simulink model "ship_location_measurements_model_dynamic"  (R2024b)
settings: Solver=VariableStepAuto  StartTime=0.0  StopTime=300  RelTol=1e-3
InitFcn:
  | dt=1;
settings Model: Creator=Noy Kirshner  LastModifiedBy=danie
settings SolverCC: AlgebraicLoopSolver=TrustRegion
settings RTWCC: GPUComputeCapability=3.5  DLArmComputeVersion=19.05

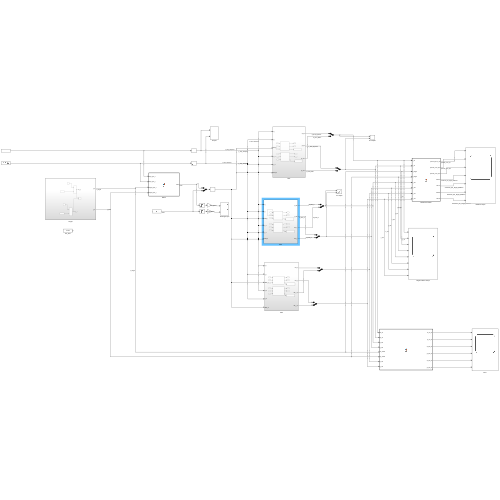
[thumbnail: Simulink's stored preview of the top-level diagram]
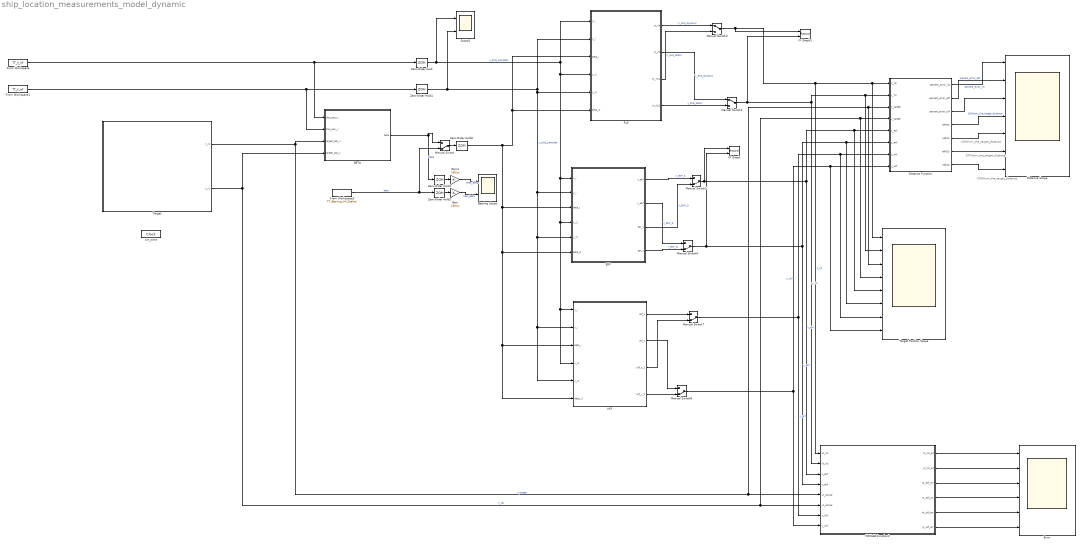
== system ship_location_measurements_model_dynamic ==
  note: -20%from_the_target_distance
  note: 20%from_the_target_distance
  note: -10%from_the_target_distance
  " Bearing Scope" : Scope  NumInputPorts=2
  " Scope1" : Scope  NumInputPorts=2
  BETA : MATLAB Function  TreatAsAtomicUnit=on
  Distance Function : MATLAB Function  TreatAsAtomicUnit=on
  Distance Scope : Scope  NumInputPorts=7
  EKF : Subsystem
  Error : Scope  NumInputPorts=6
      settings: Description=error
  From Workspace : FromWorkspace  VariableName=TT_X_inf  SampleTime=0.001
  From Workspace1 : FromWorkspace  VariableName=TT_Y_inf  SampleTime=0.001
  From Workspace3 : FromWorkspace  VariableName=TT_Bearing_Inf_Scaled
  Gain : Gain  Gain=180/pi
  Gain1 : Gain  Gain=180/pi
  MATLAB Function2 : MATLAB Function  TreatAsAtomicUnit=on
  Manual Switch{,4..7} (5 alike) : ManualSwitch  CurrentSetting=0
  Manual Switch2 : ManualSwitch
  Manual Switch3 : ManualSwitch
  RLS : Subsystem
  Target : Subsystem
  Target Position Scope : Scope  NumInputPorts=8
  UKF : Subsystem
  XY Graph : Record  FileSettingsInternal="{\"entries\":[{\"content\":{\"excelSettings\":{\"content\":{},\"type\":\"Streamout.ExcelSettings\"}},\"type\":\"Streamout.FileSettingStorage\",\"uuid\":\"\"}],\"packageUris\":[\"http:\\/\\/schema.mathworks.com\\/mf0\\/streamout_blocks\\/R2020a\"],\"version\":\"1.0\"}"  Layout=[1 1]  SignalsInternal="{\"entries\":[{\"content\":{\"signals\":[{\"content\":{\"blockPath\":[],\"dimensions\":[1],\"domain\":\"\",\"lineColor\":\"#a2142f\",\"plots\":[ 1 ],\"port\":1,\"signalID\":1,\"signalName\":\"x_ekf\"},\"type\":\"RecordBlkView.Signal\",\"uuid\":\"\"},{\"content\":{\"blockPath\":[],\"dimensions\":[1],\"domain\":\"\",\"lineColor\":\"#139fff\",\"plots\":[ 1 ],\"port\":2,\"signalID\":2,\"signalName\":\"y_ekf\"},\"type\":\"RecordBlkView.Signal\",\"uuid\":\"\"}]},\"type\":\"RecordBlkView.InputSignals\",\"uuid\":\"\"}],\"packageUris\":[\"http:\\/\\/schema.mathworks.com\\/mf0\\/streamout_blocks\\/R2020a\"],\"version\":\"1.0\"}"  VisualizationBindings="{\"xyplotplugin\":{\"info\":[{\"series\":[{\"bindingParametersList\":[{\"parameter\":\"X-Axis\",\"signalID\":1,\"signalName\":\"x_ekf\"},{\"parameter\":\"Y-Axis\",\"signalID\":2,\"signalName\":\"y_ekf\"}],\"seriesID\":0}],\"subplotID\":1}]}}"  CompatibilityTag=XY
  XY Graph1 : Record  FileSettingsInternal="{\"entries\":[{\"content\":{\"excelSettings\":{\"content\":{},\"type\":\"Streamout.ExcelSettings\"}},\"type\":\"Streamout.FileSettingStorage\",\"uuid\":\"\"}],\"packageUris\":[\"http:\\/\\/schema.mathworks.com\\/mf0\\/streamout_blocks\\/R2020a\"],\"version\":\"1.0\"}"  Layout=[1 1]  SignalsInternal="{\"entries\":[{\"content\":{\"signals\":[{\"content\":{\"blockPath\":[],\"dimensions\":[1],\"domain\":\"\",\"lineColor\":\"#a2142f\",\"plots\":[ 1 ],\"port\":1,\"signalID\":1,\"signalName\":\"x_rls\"},\"type\":\"RecordBlkView.Signal\",\"uuid\":\"\"},{\"content\":{\"blockPath\":[],\"dimensions\":[1],\"domain\":\"\",\"lineColor\":\"#139fff\",\"plots\":[ 1 ],\"port\":2,\"signalID\":2,\"signalName\":\"y_rls\"},\"type\":\"RecordBlkView.Signal\",\"uuid\":\"\"}]},\"type\":\"RecordBlkView.InputSignals\",\"uuid\":\"\"}],\"packageUris\":[\"http:\\/\\/schema.mathworks.com\\/mf0\\/streamout_blocks\\/R2020a\"],\"version\":\"1.0\"}"  VisualizationBindings="{\"xyplotplugin\":{\"info\":[{\"series\":[{\"bindingParametersList\":[{\"parameter\":\"X-Axis\",\"signalID\":1,\"signalName\":\"x_rls\"},{\"parameter\":\"Y-Axis\",\"signalID\":2,\"signalName\":\"y_rls\"}],\"seriesID\":0}],\"subplotID\":1}]}}"  CompatibilityTag=XY
  Zero-Order Hold : ZeroOrderHold  SampleTime=dt
  Zero-Order Hold1 : ZeroOrderHold
  Zero-Order Hold2 : ZeroOrderHold  SampleTime=0.1
  Zero-Order Hold3 : ZeroOrderHold
  Zero-Order Hold4 : ZeroOrderHold
  sim_time : DigitalClock
  wires:
  Manual Switch/1 -> Zero-Order Hold2/1
  From Workspace1/1 -> BETA/2(ship_pos_y), Zero-Order Hold1/1
  From Workspace/1 -> BETA/1(ship_pos_x), Zero-Order Hold/1
  Zero-Order Hold3/1 -> Gain/1
  Gain/1 -> " Bearing Scope"/2  "Mes_Beta"
  Gain1/1 -> " Bearing Scope"/1  "Theo_Beta"
  Zero-Order Hold4/1 -> Gain1/1
  BETA/1(beta) -> Manual Switch/1, Zero-Order Hold4/1  "beta"
  Target/1(x_i1) -> Target Position Scope/3, Distance Function/3(x_target), MATLAB Function2/5(xt_actual), BETA/3(target_pos_x)  "x_target"
  RLS/2(yt_rls) -> Manual Switch2/1  "Y_RLS_Dynamic"
  Distance Function/6(refH20) -> Distance Scope/6
  Distance Function/7(refL20) -> Distance Scope/7
  Distance Function/4(refH10) -> Distance Scope/4  "10%from_the_target_distance"
  MATLAB Function2/3(xt_ekf_err) -> Error/3
  Manual Switch7/1 -> Target Position Scope/7, Distance Function/7(x_ukf), MATLAB Function2/7(x_ukf)  "x_ukf"
  RLS/1(xt_rls) -> Manual Switch3/1  "X_RLS_Dynamic"
  MATLAB Function2/4(yt_ekf_err) -> Error/4
  MATLAB Function2/6(yt_ukf_err) -> Error/6
  Zero-Order Hold1/1 -> " Scope1"/2, RLS/5(y_i1), UKF/5(y_i1), UKF/2(y_i), EKF/5(y_i1), EKF/2(y_i), RLS/2(y_i)  "y_ship_sampled"
  Distance Function/3(percent_error_ukf) -> Distance Scope/3
  MATLAB Function2/5(xt_ukf_err) -> Error/5
  MATLAB Function2/2(yt_rls_err) -> Error/2
  UKF/4(ukf_y_2) -> Manual Switch6/2
  Manual Switch4/1 -> XY Graph/2, Target Position Scope/6, Distance Function/6(y_ekf), MATLAB Function2/4(y_ekf)  "y_ekf"
  UKF/2(ukf_y) -> Manual Switch6/1
  MATLAB Function2/1(xt_rls_err) -> Error/1
  Distance Function/1(percent_error_rls) -> Distance Scope/1  "percent_error_rls"
  EKF/2(y_ekf) -> Manual Switch4/1  "Y_EKF_S"
  Manual Switch3/1 -> XY Graph1/1, MATLAB Function2/1(xt_rls), Distance Function/1(x_rls), Target Position Scope/1  "x_rls"
  Target/2(y_i1) -> Target Position Scope/4, Distance Function/4(y_target), MATLAB Function2/6(yt_actual), BETA/4(target_pos_y)  "y_tar"
  Zero-Order Hold/1 -> " Scope1"/1, RLS/1(x_i), EKF/1(x_i), UKF/4(x_i1), UKF/1(x_i), EKF/4(x_i1), RLS/4(x_i1)  "x_ship_sampled"
  Manual Switch6/1 -> Target Position Scope/8, Distance Function/8(y_ukf), MATLAB Function2/8(y_ukf)  "y_ukf"
  Manual Switch2/1 -> XY Graph1/2, Distance Function/2(y_rls), Target Position Scope/2, MATLAB Function2/2(yt_rls)  "y_rls"
  UKF/1(ukf_x) -> Manual Switch7/1
  Distance Function/2(percent_error_ekf) -> Distance Scope/2  "precent_error_ekf"
  RLS/4(yt_rls1) -> Manual Switch2/2  "Y_RLS_Static"
  UKF/3(ukf_x_2) -> Manual Switch7/2
  EKF/1(x_ekf) -> Manual Switch5/1  "X_EKF_S"
  RLS/3(xt_rls1) -> Manual Switch3/2  "X_RLS_Static"
  Manual Switch5/1 -> XY Graph/1, MATLAB Function2/3(x_ekf), Target Position Scope/5, Distance Function/5(x_ekf)  "x_ekf"
  EKF/4(est_y) -> Manual Switch4/2  "Y_EKF_D"
  Distance Function/5(refL10) -> Distance Scope/5
  EKF/3(est_x) -> Manual Switch5/2  "X_EKF_D"
  Zero-Order Hold2/1 -> UKF/6(beta_i1), UKF/3(beta_i), EKF/6(beta_i1), EKF/3(beta_i), RLS/6(beta_i1), RLS/3(beta_i)
  From Workspace3/1 -> Manual Switch/2, Zero-Order Hold3/1  "beta"

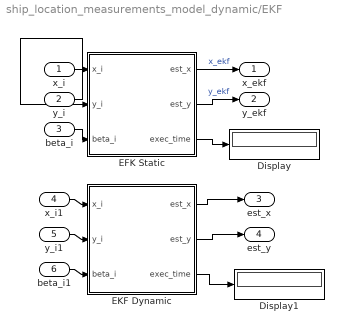
== system ship_location_measurements_model_dynamic/EKF ==
  x_i : Inport
  y_i : Inport  Port=2
  beta_i : Inport  Port=3
  x_i1 : Inport  Port=4
  y_i1 : Inport  Port=5
  beta_i1 : Inport  Port=6
  Display : Display
  Display1 : Display
  EFK Static : MATLAB Function  TreatAsAtomicUnit=on
  EKF Dynamic : MATLAB Function  TreatAsAtomicUnit=on
  x_ekf : Outport
  y_ekf : Outport  Port=2
  est_x : Outport  Port=3
  est_y : Outport  Port=4
  wires:
  y_i/1 -> EFK Static/2(y_i)
  EKF Dynamic/2(est_y) -> est_y/1
  x_i/1 -> EFK Static/1(x_i)
  x_i1/1 -> EKF Dynamic/1(x_i)
  y_i1/1 -> EKF Dynamic/2(y_i)
  EFK Static/2(est_y) -> y_ekf/1  "y_ekf"
  EFK Static/1(est_x) -> x_ekf/1  "x_ekf"
  beta_i/1 -> EFK Static/3(beta_i)
  beta_i1/1 -> EKF Dynamic/3(beta_i)
  EKF Dynamic/1(est_x) -> est_x/1
  EFK Static/3(exec_time) -> Display/1
  EKF Dynamic/3(exec_time) -> Display1/1

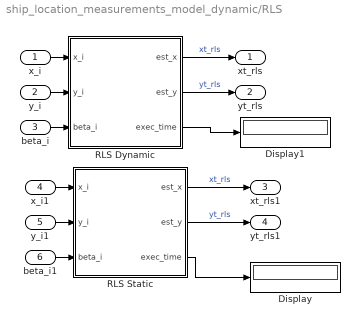
== system ship_location_measurements_model_dynamic/RLS ==
  x_i : Inport
  y_i : Inport  Port=2
  beta_i : Inport  Port=3
  x_i1 : Inport  Port=4
  y_i1 : Inport  Port=5
  beta_i1 : Inport  Port=6
  Display : Display
  Display1 : Display
  RLS Dynamic : MATLAB Function  TreatAsAtomicUnit=on
  RLS Static : MATLAB Function  TreatAsAtomicUnit=on
  xt_rls : Outport
  yt_rls : Outport  Port=2
  xt_rls1 : Outport  Port=3
  yt_rls1 : Outport  Port=4
  wires:
  RLS Static/1(est_x) -> xt_rls1/1  "xt_rls"
  beta_i/1 -> RLS Dynamic/3(beta_i)
  y_i1/1 -> RLS Static/2(y_i)
  x_i1/1 -> RLS Static/1(x_i)
  beta_i1/1 -> RLS Static/3(beta_i)
  x_i/1 -> RLS Dynamic/1(x_i)
  RLS Static/2(est_y) -> yt_rls1/1  "yt_rls"
  y_i/1 -> RLS Dynamic/2(y_i)
  RLS Dynamic/1(est_x) -> xt_rls/1  "xt_rls"
  RLS Dynamic/2(est_y) -> yt_rls/1  "yt_rls"
  RLS Static/3(exec_time) -> Display/1
  RLS Dynamic/3(exec_time) -> Display1/1

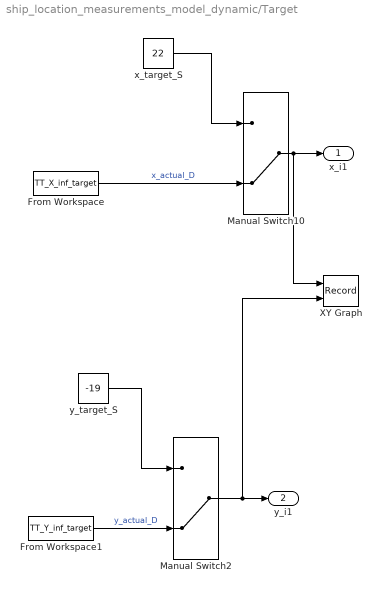
== system ship_location_measurements_model_dynamic/Target ==
  From Workspace : FromWorkspace  VariableName=TT_X_inf_target
  From Workspace1 : FromWorkspace  VariableName=TT_Y_inf_target
  Manual Switch10 : ManualSwitch  CurrentSetting=0
  Manual Switch2 : ManualSwitch  CurrentSetting=0
  XY Graph : Record  FileSettingsInternal="{\"entries\":[{\"content\":{\"excelSettings\":{\"content\":{},\"type\":\"Streamout.ExcelSettings\"}},\"type\":\"Streamout.FileSettingStorage\",\"uuid\":\"\"}],\"packageUris\":[\"http:\\/\\/schema.mathworks.com\\/mf0\\/streamout_blocks\\/R2020a\"],\"version\":\"1.0\"}"  Layout=[1 1]  SignalsInternal="{\"entries\":[{\"content\":{\"signals\":[{\"content\":{\"blockPath\":[],\"dimensions\":[1],\"domain\":\"\",\"lineColor\":\"#a2142f\",\"plots\":[ 1 ],\"port\":1,\"signalID\":1,\"signalName\":\"Manual Switch10\"},\"type\":\"RecordBlkView.Signal\",\"uuid\":\"\"},{\"content\":{\"blockPath\":[],\"dimensions\":[1],\"domain\":\"\",\"lineColor\":\"#139fff\",\"plots\":[ 1 ],\"port\":2,\"signalID\":2,\"signalName\":\"Manual Switch2\"},\"type\":\"RecordBlkView.Signal\",\"uuid\":\"\"}]},\"type\":\"RecordBlkView.InputSignals\",\"uuid\":\"\"}],\"packageUris\":[\"http:\\/\\/schema.mathworks.com\\/mf0\\/streamout_blocks\\/R2020a\"],\"version\":\"1.0\"}"  VisualizationBindings="{\"xyplotplugin\":{\"info\":[{\"series\":[{\"bindingParametersList\":[{\"parameter\":\"X-Axis\",\"signalID\":1,\"signalName\":\"Manual Switch10\"},{\"parameter\":\"Y-Axis\",\"signalID\":2,\"signalName\":\"Manual Switch2\"}],\"seriesID\":0}],\"subplotID\":1}]}}"  CompatibilityTag=XY
  x_target_S : Constant  Value=22
  y_target_S : Constant  Value=-19
  x_i1 : Outport
  y_i1 : Outport  Port=2
  wires:
  From Workspace1/1 -> Manual Switch2/2  "y_actual_D"
  Manual Switch10/1 -> XY Graph/1, x_i1/1
  x_target_S/1 -> Manual Switch10/1
  y_target_S/1 -> Manual Switch2/1
  From Workspace/1 -> Manual Switch10/2  "x_actual_D"
  Manual Switch2/1 -> XY Graph/2, y_i1/1

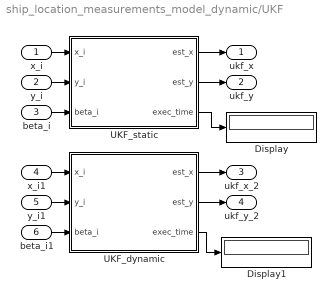
== system ship_location_measurements_model_dynamic/UKF ==
  x_i : Inport
  y_i : Inport  Port=2
  beta_i : Inport  Port=3
  x_i1 : Inport  Port=4
  y_i1 : Inport  Port=5
  beta_i1 : Inport  Port=6
  Display : Display
  Display1 : Display
  UKF_dynamic : MATLAB Function  TreatAsAtomicUnit=on
  UKF_static : MATLAB Function  TreatAsAtomicUnit=on
  ukf_x : Outport
  ukf_y : Outport  Port=2
  ukf_x_2 : Outport  Port=3
  ukf_y_2 : Outport  Port=4
  wires:
  UKF_dynamic/1(est_x) -> ukf_x_2/1
  UKF_static/2(est_y) -> ukf_y/1
  beta_i/1 -> UKF_static/3(beta_i)
  x_i/1 -> UKF_static/1(x_i)
  x_i1/1 -> UKF_dynamic/1(x_i)
  UKF_static/1(est_x) -> ukf_x/1
  y_i1/1 -> UKF_dynamic/2(y_i)
  y_i/1 -> UKF_static/2(y_i)
  UKF_dynamic/2(est_y) -> ukf_y_2/1
  beta_i1/1 -> UKF_dynamic/3(beta_i)
  UKF_static/3(exec_time) -> Display/1
  UKF_dynamic/3(exec_time) -> Display1/1

== matlab function ship_location_measurements_model_dynamic/UKF/UKF_static ==
  settings: updateMethod=DISCRETE
  data: x_i input; est_x output; y_i input; beta_i input; est_y output; exec_time output
function [est_x, est_y, exec_time] = ukf_fcn(x_i, y_i, beta_i)

persistent X_i P Q R lambda alpha beta nx

% Initialize execution time variable  
exec_time = 0; % Ensures fixed-size output for Simulink compatibility  

% Start timing  
coder.extrinsic('tic', 'toc'); % Allows tic/toc in Simulink  
tStart = tic; % Capture start time 

if isempty(P)
    nx = 6; % State dimension
    P = 1000* eye(nx); % Covariance matrix initialization (6x6)
    Q = 10 * diag([0.01, 0.01, 1, 0.01, 1, 0.01]); % Process noise covariance (6x6)
    R = diag([1, 1, 100]); % Measurement noise covariance (3x3)
    
    % UKF parameters
    alpha = 1e-3; % Spread of sigma points
    beta = 2; % Optimal for Gaussian distribution
    lambda = alpha^2 * (nx + 1) - nx; % Scaling parameter
end

if isempty(X_i)
    X_i = zeros(nx, 1); % State vector initialization (6x1)
end

dt = 0.01; % Sample time variable

% Weights for UKF
Wm = [lambda / (nx + lambda); repmat(1 / (2 * (nx + lambda)), 2 * nx, 1)];
Wc = Wm;
Wc(1) = Wc(1) + (1 - alpha^2 + beta);

% Generate sigma points
sigma_points = generate_sigma_points(X_i, P, lambda);

% Prediction Step
predicted_sigma_points = process_model(sigma_points, dt);
[X_pred, P_pred] = compute_mean_and_covariance(predicted_sigma_points, Wm, Wc, Q);

% Measurement Step
measured_sigma_points = measurement_model(predicted_sigma_points, beta_i);
[y_pred, Pyy] = compute_mean_and_covariance(measured_sigma_points, Wm, Wc, R);

% Cross covariance
Pxy = compute_cross_covariance(predicted_sigma_points, measured_sigma_points, X_pred, y_pred, Wc);

% Kalman Gain
K = Pxy / Pyy;

% Measurement update
meas = [x_i; y_i; 0]; % Measurements
resid = meas - y_pred; % Residual
X_i = X_pred + K * resid; % State update
P = P_pred - K * Pyy * K'; % Covariance update

% Output estimated position
est_x = X_i(1); % x_t estimation
est_y = X_i(2); % y_t estimation

% Stop timing  
exec_time = toc(tStart); % Store execution time

end

%% Helper Functions

% Generate sigma points
function sigma_points = generate_sigma_points(mean, covariance, lambda)
    nx = length(mean);
    S = chol((nx + lambda) * covariance, 'lower');
    sigma_points = [mean, bsxfun(@plus, mean, S), bsxfun(@minus, mean, S)];
end

% Process model
function predicted_sigma_points = process_model(sigma_points, dt)
    F = [1 0 0 0 0 0;
         0 1 0 0 0 0;
         0 0 1 dt 0 0;
         0 0 0 1 0 0;
         0 0 0 0 1 dt;
         0 0 0 0 0 1]; % Process model matrix
    predicted_sigma_points = F * sigma_points;
end

% Measurement model
function measured_sigma_points = measurement_model(sigma_points, beta_i)
    H = [0 0 1 0 0 0;
         0 0 0 0 1 0;
         sin(beta_i) -cos(beta_i) -sin(beta_i) 0 cos(beta_i) 0]; % Measurement model matrix
    measured_sigma_points = H * sigma_points;
end

% Compute mean and covariance
function [mean_out, covariance] = compute_mean_and_covariance(sigma_points, Wm, Wc, noise_cov)
    mean_out = sigma_points * Wm; % Weighted mean
    diff = bsxfun(@minus, sigma_points, mean_out);
    covariance = diff * diag(Wc) * diff' + noise_cov; % Weighted covariance
end

% Compute cross covariance
function Pxy = compute_cross_covariance(predicted_sigma_points, measured_sigma_points, X_pred, y_pred, Wc)
    diff_x = bsxfun(@minus, predicted_sigma_points, X_pred);
    diff_y = bsxfun(@minus, measured_sigma_points, y_pred);
    Pxy = diff_x * diag(Wc) * diff_y'; % Cross covariance
end

== matlab function ship_location_measurements_model_dynamic/UKF/UKF_dynamic ==
  settings: updateMethod=DISCRETE
  data: x_i input; est_x output; y_i input; beta_i input; est_y output; exec_time output
function [est_x, est_y, exec_time] = ukf_dynamic_fcn(x_i, y_i, beta_i)

persistent X_i P Q R lambda alpha beta nx

% Initialize execution time variable  
exec_time = 0; % Ensures fixed-size output for Simulink compatibility  

% Start timing  
coder.extrinsic('tic', 'toc'); % Allows tic/toc in Simulink  
tStart = tic; % Capture start time  

if isempty(P)
    nx = 8; % State dimension for dynamic model
    P = 10 * eye(nx); % Covariance matrix initialization (8x8)
    Q =0.1* diag([1, 0.01, 1, 0.01, 1, 0.01, 1, 0.01]); % Process noise covariance (8x8)
    R = diag([1, 1, 400]); % Measurement noise covariance (3x3)
    
    % UKF parameters
    alpha = 1e-3; % Spread of sigma points
    beta = 2; % Optimal for Gaussian distribution
    lambda = alpha^2 * (nx + 1) - nx; % Scaling parameter
end

if isempty(X_i)
    X_i = zeros(nx, 1); % State vector initialization (8x1)
end

dt = 0.001; % Sample time variable

% Weights for UKF
Wm = [lambda / (nx + lambda); repmat(1 / (2 * (nx + lambda)), 2 * nx, 1)];
Wc = Wm;
Wc(1) = Wc(1) + (1 - alpha^2 + beta);

% Generate sigma points
sigma_points = generate_sigma_points(X_i, P, lambda);

% Prediction Step
predicted_sigma_points = process_model(sigma_points, dt);
[X_pred, P_pred] = compute_mean_and_covariance(predicted_sigma_points, Wm, Wc, Q);

% Measurement Step
measured_sigma_points = measurement_model(predicted_sigma_points, beta_i);
[y_pred, Pyy] = compute_mean_and_covariance(measured_sigma_points, Wm, Wc, R);

% Cross covariance
Pxy = compute_cross_covariance(predicted_sigma_points, measured_sigma_points, X_pred, y_pred, Wc);

% Kalman Gain
K = Pxy / Pyy;

% Measurement update
meas = [x_i; y_i; 0]; % Measurements
resid = meas - y_pred; % Residual
X_i = X_pred + K * resid; % State update
P = P_pred - K * Pyy * K'; % Covariance update

% Output estimated position
est_x = X_i(1); % x_t estimation
est_y = X_i(3); % y_t estimation

% Stop timing  
exec_time = toc(tStart); % Store execution time  

end

%% Helper Functions

% Generate sigma points
function sigma_points = generate_sigma_points(mean, covariance, lambda)
    nx = length(mean);
    S = chol((nx + lambda) * covariance, 'lower');
    sigma_points = [mean, bsxfun(@plus, mean, S), bsxfun(@minus, mean, S)];
end

% Process model
function predicted_sigma_points = process_model(sigma_points, dt)
    F = [1 dt 0 0 0 0 0 0; 
         0 1 0 0 0 0 0 0; 
         0 0 1 dt 0 0 0 0; 
         0 0 0 1 0 0 0 0; 
         0 0 0 0 1 dt 0 0; 
         0 0 0 0 0 1 0 0; 
         0 0 0 0 0 0 1 dt; 
         0 0 0 0 0 0 0 1]; % Process model matrix for dynamic system
    predicted_sigma_points = F * sigma_points;
end

% Measurement model
function measured_sigma_points = measurement_model(sigma_points, beta_i)
    H = [0 0 0 0 1 0 0 0;
         0 0 0 0 0 0 1 0;
         sin(beta_i) 0 -cos(beta_i) 0 -sin(beta_i) 0 cos(beta_i) 0]; % Measurement model matrix
    measured_sigma_points = H * sigma_points;
end

% Compute mean and covariance
function [mean_out, covariance] = compute_mean_and_covariance(sigma_points, Wm, Wc, noise_cov)
    mean_out = sigma_points * Wm; % Weighted mean
    diff = bsxfun(@minus, sigma_points, mean_out);
    covariance = diff * diag(Wc) * diff' + noise_cov; % Weighted covariance
end

% Compute cross covariance
function Pxy = compute_cross_covariance(predicted_sigma_points, measured_sigma_points, X_pred, y_pred, Wc)
    diff_x = bsxfun(@minus, predicted_sigma_points, X_pred);
    diff_y = bsxfun(@minus, measured_sigma_points, y_pred);
    Pxy = diff_x * diag(Wc) * diff_y'; % Cross covariance
end

== matlab function ship_location_measurements_model_dynamic/BETA ==
  data: ship_pos_x input; beta output; ship_pos_y input; target_pos_x input; target_pos_y input
function beta = fcn(ship_pos_x,ship_pos_y,target_pos_x,target_pos_y)
% Calculation of the horizontal distance (dx) between the target and the ship

% Calculation of the horizontal distance (dx) between the target and the ship
dx = target_pos_x - ship_pos_x;

% Calculation of the vertical distance (dy) between the target and the ship
dy = target_pos_y - ship_pos_y;

% atan2(dy, dx) returns the angle in radians in the range \[-pi, pi]
beta = atan2(dy,dx);
end

== matlab function ship_location_measurements_model_dynamic/EKF/EFK Static ==
  settings: updateMethod=DISCRETE
  data: x_i input; est_x output; y_i input; beta_i input; est_y output; exec_time output
function [est_x, est_y, exec_time] = ekf_fcn(x_i, y_i, beta_i)

persistent X_i P Q R

% Initialize execution time variable  
exec_time = 0; % Ensures fixed-size output for Simulink compatibility  

% Start timing  
coder.extrinsic('tic', 'toc'); % Allows tic/toc in Simulink  
tStart = tic; % Capture start time

if isempty(P)
    P = 1000*eye(6); % Covariance matrix initialization (6x6)
    Q = 10*diag([0.01, 0.01, 1, 0.01, 1, 0.01]); % Process noise covariance initialization (6x6)
    R = diag([1, 1, 100]); % Measurement noise covariance initialization (3x3)
end

if isempty(X_i)
    X_i = zeros(6, 1); % State vector initialization (6x1)
end

dt = 0.01; % Sample time variable
F = [1 0 0 0 0 0 ; 0 1 0 0 0 0 ; 0 0 1 dt 0 0 ; 0 0 0 1 0 0 ; 0 0 0 0 1 dt ; 0 0 0 0 0 1]; % Process Jacobian (6x6)
H = [0 0 1 0 0 0 ; 0 0 0 0 1 0 ; sin(beta_i) -cos(beta_i) -sin(beta_i) 0 cos(beta_i) 0]; % Measurement Jacobian (3x6)

% Prediction Step
X_i = F*X_i; % Process Model
meas = [x_i ; y_i ; 0]; % Measurements
y_hat = H*X_i; % Measurement Model
P = F*P*F' + Q; % Covariance matrix

% Update Step
resid = meas - y_hat; % Measurement residual
K = P*H'/(H*P*H' + R); % Kalman gain
X_i = X_i + K*resid; % State vector update
P = (eye(6) - K*H)*P; % Covariance matrix update

% Output estimated position
est_x = X_i(1); % x_t estimation
est_y = X_i(2); % y_t estimation

% Stop timing  
exec_time = toc(tStart); % Store execution time  

end

== matlab function ship_location_measurements_model_dynamic/EKF/EKF Dynamic ==
  settings: updateMethod=DISCRETE
  data: x_i input; est_x output; y_i input; beta_i input; est_y output; exec_time output
function [est_x, est_y, exec_time] = ekf_fcn(x_i, y_i, beta_i)

persistent X_i P Q R

% Initialize execution time variable  
exec_time = 0; % Ensures fixed-size output for Simulink compatibility  

% Start timing  
coder.extrinsic('tic', 'toc'); % Allows tic/toc in Simulink  
tStart = tic; % Capture start time  

if isempty(P)
    P = 10*eye(8); % Covariance matrix initialization (8x8)
    Q = 0.1*diag([1, 0.01, 1, 0.01, 1, 0.01, 1, 0.01]); % Process noise covariance initialization (8x8)
    R = diag([1, 1, 400]); % Measurement noise covariance initialization (3x3)
end
 
if isempty(X_i)
    X_i = zeros(8, 1); % State vector initialization (8x1)
end

dt = 0.001; % Sample time variable
F = [1 dt 0 0 0 0 0 0 ; 0 1 0 0 0 0 0 0 ; 0 0 1 dt 0 0 0 0 ; 0 0 0 1 0 0 0 0 ; 0 0 0 0 1 dt 0 0 ; 0 0 0 0 0 1 0 0 ; 0 0 0 0 0 0 1 dt ; 0 0 0 0 0 0 0 1]; % Process Jacobian (8x8)
H = [0 0 0 0 1 0 0 0 ; 0 0 0 0 0 0 1 0 ; sin(beta_i) 0 -cos(beta_i) 0 -sin(beta_i) 0 cos(beta_i) 0]; % Measurement Jacobian (3x8)

% Prediction Step
X_i = F*X_i; % Process Model
meas = [x_i ; y_i ; 0]; % Measurements
y_hat = H*X_i; % Measurement Model
P = F*P*F' + Q; % Covariance matrix

% Update Step
resid = meas - y_hat; % Measurement residual
K = P*H'/(H*P*H' + R); % Kalman gain
X_i = X_i + K*resid; % State vector update
P = (eye(8) - K*H)*P; % Covariance matrix update

% Output estimated position
est_x = X_i(1); % x_t estimation
est_y = X_i(3); % y_t estimation

% Stop timing  
exec_time = toc(tStart); % Store execution time  

end

== matlab function ship_location_measurements_model_dynamic/RLS/RLS Dynamic ==
  settings: updateMethod=DISCRETE
  data: x_i input; est_x output; y_i input; beta_i input; est_y output; exec_time output
function [est_x, est_y, exec_time] = fcn(x_i, y_i, beta_i) 
% FCN Perform recursive least squares (RLS) algorithm with a forgetting factor to estimate
% the position of a target based on noisy measurements and angular data.
% Outputs: est_x - Estimated x-coordinate of the target and est_y - Estimated y-coordinate of the target

% Declartion of the persistent variables 
persistent P X_i lambda lambda_initial

% Initialize execution time variable  
exec_time = 0; % Ensures fixed-size output for Simulink compatibility  

% Start timing  
coder.extrinsic('tic', 'toc'); % Allows tic/toc in Simulink  
tStart = tic; % Capture start time 

% Initialization of the persistent variables on the first function call
if isempty(P)
    P = 1*eye(2);  % Initialization of the covariance matrix as a 2x2 identity matrix
    lambda_initial = 0.98; % Initial forgetting factor
    lambda = 1; % Initial adaptive forgetting factor
end

if isempty(X_i)
    X_i = zeros(2, 1);  % Initialization of the state vector (X) as a 2x1 zero vector
end

% Update the observation model
phi_i = [-sin(beta_i); cos(beta_i)];  % The observation vector (phi)
z_i = y_i * cos(beta_i) - x_i * sin(beta_i);  % The measurement scalar (z)

% The estimation error
e = z_i - phi_i' * X_i;  % Error between measurement and model prediction

% The weighting vector
g_k = P * phi_i / (lambda + phi_i' * P * phi_i);  

% Updating the state vector with the new measurement
X_i = X_i + g_k * e;  % Recursive state update

% Updating the covariance matrix using the forgetting factor
P = (1 / lambda) * (P - g_k * phi_i' * P);  % Update covariance matrix

% Adapt the forgetting factor
lambda = lambda_initial * lambda + (1 - lambda_initial);

%The estimated position from the updated state vector
est_x = X_i(1);  % Estimated x-coordinate
est_y = X_i(2);  % Estimated y-coordinate

% Stop timing  
exec_time = toc(tStart); % Store execution time  

end

== matlab function ship_location_measurements_model_dynamic/RLS/RLS Static ==
  settings: updateMethod=DISCRETE
  data: x_i input; est_x output; y_i input; beta_i input; est_y output; exec_time output
function [est_x, est_y, exec_time] = fcn(x_i, y_i, beta_i)  
% FCN Perform recursive estimation for position using a RLS algorithm  
% Outputs:  
% - est_x: Estimated x-coordinate  
% - est_y: Estimated y-coordinate  
% - exec_time: Execution time (fixed-size double for Simulink compatibility)  

% Declare persistent variables  
persistent Q P X_i  

% Initialize execution time variable  
exec_time = 0; % Explicitly define as a scalar double (important for Simulink)  

% Start timing  
coder.extrinsic('tic', 'toc'); % Allow tic/toc in Simulink  
tStart = tic; % Capture start time  

% Initialization of the covariance matrix P on the first function call  
if isempty(P)  
    P = 1000 * eye(2); % Start with a large initial uncertainty  
end  

if isempty(Q)  
    Q = 0 * eye(2); % No process noise initially  
end  

% Initialization of the state vector X_i on the first function call  
if isempty(X_i)  
    X_i = zeros(2, 1); % Start with zero state  
end  

% Observation vector based on the angle beta_i  
phi_i = [-sin(beta_i); cos(beta_i)]; % The observation model  

% Measurement scalar z_i derived from the input coordinates and angle  
z_i = y_i * cos(beta_i) - x_i * sin(beta_i);  

% The estimation error  
e = z_i - phi_i' * X_i; % Prediction error  

% The weighting vector  
g_k = P * phi_i / (1 + phi_i' * P * phi_i);  

% Update the state vector with the new measurement  
X_i = X_i + g_k * e;  

% Update the covariance matrix  
P = P - g_k * phi_i' * P + Q;  

% Extract estimated position  
est_x = X_i(1);  
est_y = X_i(2);  

% End timing and store execution time  
exec_time = toc(tStart); % Ensure exec_time is a fixed-size double  

end

== matlab function ship_location_measurements_model_dynamic/Distance Function ==
  data: percent_error_rls output; percent_error_ekf output; percent_error_ukf output; x_rls input; refH10 output; y_rls input; x_target input; y_target input; x_ekf input; y_ekf input; x_ukf input; y_ukf input; refL10 output; refH20 output; refL20 output
function [percent_error_rls,percent_error_ekf,percent_error_ukf,refH10, refL10,refH20, refL20]= fcn(x_rls,y_rls,x_target,y_target, x_ekf, y_ekf,x_ukf, y_ukf)

% Circle center
xc = 5.5;
yc = 1.5;

% Circle radius
r = 2.0;  
% Normalized distances (radial distance from center)
distance_target = sqrt((x_target - xc)^2 + (y_target - yc)^2) / r;
distance_rls    = sqrt((x_rls    - xc)^2 + (y_rls    - yc)^2) / r;
distance_ekf    = sqrt((x_ekf    - xc)^2 + (y_ekf    - yc)^2) / r;
distance_ukf    = sqrt((x_ukf    - xc)^2 + (y_ukf    - yc)^2) / r;

% Percentage errors relative to the target
percent_error_rls = (abs(distance_rls - distance_target) / distance_target) * 100;
percent_error_ekf = (abs(distance_ekf - distance_target) / distance_target) * 100;
percent_error_ukf = (abs(distance_ukf - distance_target) / distance_target) * 100;

% Reference bands (±10%, ±20% of target normalized distance)
refH10 = 0.1 * distance_target;
refL10 = -0.1 * distance_target;
refH20 = 0.2 * distance_target;
refL20 = -0.2 * distance_target;
end

== matlab function ship_location_measurements_model_dynamic/MATLAB Function2 ==
  data: xt_rls input; xt_rls_err output; yt_rls_err output; yt_rls input; x_ekf input; y_ekf input; xt_actual input; yt_actual input; xt_ekf_err output; yt_ekf_err output; x_ukf input; y_ukf input; xt_ukf_err output; yt_ukf_err output
function [xt_rls_err,yt_rls_err,xt_ekf_err,yt_ekf_err,xt_ukf_err,yt_ukf_err]   = fcn(xt_rls,yt_rls, x_ekf, y_ekf,xt_actual,yt_actual,x_ukf,y_ukf)
% FCN Computes the percentage error for RLS and EKF position estimates

% The percentage error for RLS estimates:
xt_rls_err = ((xt_rls - xt_actual)/xt_actual)*100;
yt_rls_err = ((yt_rls - yt_actual)/yt_actual)*100;

% The percentage error for EKF estimates:
xt_ekf_err = ((x_ekf - xt_actual)/xt_actual)*100;
yt_ekf_err = ((y_ekf - yt_actual)/yt_actual)*100;

xt_ukf_err = ((x_ukf - xt_actual)/xt_actual)*100;
yt_ukf_err = ((y_ukf - yt_actual)/yt_actual)*100;
